simulink model "Lab3_Crazyflie_Task1"  (R2020a)
settings: Solver=FixedStepAuto  StartTime=0.0  StopTime=inf  MaxStep=0.1  RelTol=1e-3  EnableMultiTasking=on
PreLoadFcn:
  | % load parameters of the default quadrotor
  | disp('Quadrotor parameters loaded by PreLoadFcn')
  | mdl_quadrotor
undefined symbols (not defined in the file or in its folder): Pitch, Roll, rot2, Thrust, YawRate
libraries: robotlib x3, simulink x2
settings Model: Creator=corkep  LastModifiedBy=Pablo
settings DataIOCC: LimitDataPoints=on  ReturnWorkspaceOutputs=off
settings OptimizationCC: EnhancedBackFolding=on  PassReuseOutputArgsAs=Individual arguments  ExpressionDepthLimit=2147483647  ZeroExternalMemoryAtStartup=off  ZeroInternalMemoryAtStartup=off  MaxStackSize=64  OptimizeBlockOrder=speed  DifferentSizesBufferReuse=on  OptimizationCustomize=off  EfficientTunableParamExpr=on
settings DebuggingCC: UnderspecifiedInitializationDetection=Classic  MergeDetectMultiDrivingBlocksExec=none  SolverPrmCheckMsg=warning  ParameterTunabilityLossMsg=error  AllowSymbolicDim=off  StateNameClashWarn=warning  SFUnexpectedBacktrackingDiag=warning  SFNoUnconditionalDefaultTransitionDiag=warning  SFExecutionAtInitializationDiag=none  ArithmeticOperatorsInVariantConditions=warning
settings HardwareCC: ProdBitPerPointer=32  ProdBitPerSizeT=32  ProdBitPerPtrDiffT=32  ProdLargestAtomicFloat=None  ProdIntDivRoundTo=Undefined  ProdEndianess=Unspecified  ProdWordSize=32  ProdHWDeviceType=Generic->Unspecified (assume 32-bit Generic)  UseEmbeddedCoderFeatures=off
settings ModelReferenceCC: PropagateSignalLabelsOutOfModel=off
settings SFSimCC: SimUseLocalCustomCode=off  MATLABDynamicMemAlloc=off  CustomCodeUndefinedFunction=UseInterfaceOnly
settings RTWCC: SystemTargetFile=ert.tlc  HardwareBoard=Robot Operating System (ROS)  TemplateMakefile=ert_default_tmf  RTWUseLocalCustomCode=off  Toolchain=Catkin  TargetLang=C++
settings CodeAppCC: ForceParamTrailComments=on  IgnoreCustomStorageClasses=off  OperatorAnnotations=on  SimulinkDataObjDesc=on  SFDataObjDesc=on  InsertBlockDesc=on
settings ERTTargetCC: SupportNonInlinedSFcns=on
settings ConfigComp: CovMetricSettings=dw  CovHtmlReporting=on  CovSaveCumulativeToWorkspaceVar=on  CovSaveSingleToWorkspaceVar=on  CovExternalEMLEnable=off  CovSFcnEnable=off

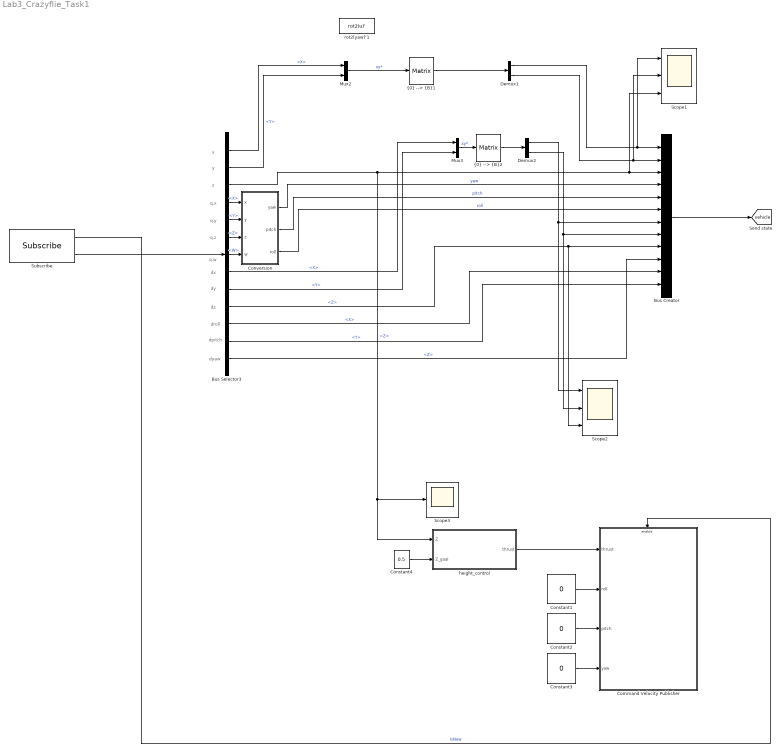
== system Lab3_Crazyflie_Task1 ==
  note: dyaw
  note: dpitch
  note: droll
  note: dz
  note: dy
  note: dx
  note: x
  note: y
  note: z
  note: q.x
  note: q.y
  note: q.z
  note: q.w
  Bus Creator : BusCreator  Inputs=12
  Bus Selector3 : BusSelector  OutputSignals=Pose.Pose.Position.X,Pose.Pose.Position.Y,Pose.Pose.Position.Z,Pose.Pose.Orientation.X,Pose.Pose.Orientation.Y,Pose.Pose.Orientation.Z,Pose.Pose.Orientation.W,Twist.Twist.Linear.X,Twist.Twist.Linear.Y,Twist.Twist.Linear.Z,Twist.Twist.Angular.X,Twist.Twist.Angular.Y,Twist.Twist.Angular.Z
  Command Velocity Publisher : Subsystem
  Constant1 : Constant  Value=0
  Constant2 : Constant  Value=0
  Constant3 : Constant  Value=0
  Constant4 : Constant  Value=0.5
  Conversion : MATLAB Function  TreatAsAtomicUnit=on
  Demux1 : Demux  Outputs=2
  Demux2 : Demux  Outputs=2
  Mux2 : Mux  Inputs=2
  Mux3 : Mux  Inputs=2
  Scope1 : Scope  NumInputPorts=3
  Scope2 : Scope  NumInputPorts=3
  Scope3 : Scope
  Subscribe : robotlib/Subscribe  topicSource=Select from ROS network  topic=/crazyflie2/ground_truth/odometry  messageType=nav_msgs/Odometry  sampleTime=-1  messageQueueLength=51
  height_control : Subsystem
  rot2(yaw)'1 : MATLABFcn  MATLABFcn=rot2(u)'  OutputDimensions=[2 2]  Output1D=off
  "{0} --> {B}1" : Product  Inputs=1  Multiplication=Matrix(*)  RndMeth=Zero
  "{0} --> {B}2" : Product  Inputs=1  Multiplication=Matrix(*)  RndMeth=Zero
  tag scope: vehicle=global
  wires:
  Bus Selector3/11 -> Bus Creator/11  "<X>"
  Bus Selector3/13 -> Bus Creator/10  "<Z>"
  Conversion/1(yaw) -> Bus Creator/4  "yaw"
  Bus Selector3/10 -> Bus Creator/9, Scope2/3  "<Z>"
  Bus Selector3/9 -> Mux3/2  "<Y>"
  Bus Selector3/8 -> Mux3/1  "<X>"
  Conversion/2(pitch) -> Bus Creator/5  "pitch"
  Bus Selector3/3 -> height_control/1(Z), Scope3/1, Scope1/3, Bus Creator/3  "<Z>"
  Bus Creator/1 -> [vehicle]
  Bus Selector3/12 -> Bus Creator/12  "<Y>"
  Conversion/3(roll) -> Bus Creator/6  "roll"
  Subscribe/2 -> Bus Selector3/1
  Bus Selector3/4 -> Conversion/1(x)  "<X>"
  Bus Selector3/5 -> Conversion/2(y)  "<Y>"
  Bus Selector3/6 -> Conversion/3(z)  "<Z>"
  Bus Selector3/7 -> Conversion/4(w)  "<W>"
  Subscribe/1 -> Command Velocity Publisher/Enable  "IsNew"
  Mux2/1 -> "{0} --> {B}1"/1  "xy*"
  "{0} --> {B}1"/1 -> Demux1/1
  "{0} --> {B}2"/1 -> Demux2/1
  Mux3/1 -> "{0} --> {B}2"/1  "xy*"
  Demux1/1 -> Bus Creator/1, Scope1/1
  Demux1/2 -> Bus Creator/2, Scope1/2
  Bus Selector3/1 -> Mux2/1  "<X>"
  Bus Selector3/2 -> Mux2/2  "<Y>"
  Demux2/1 -> Bus Creator/7, Scope2/1
  Demux2/2 -> Bus Creator/8, Scope2/2
  height_control/1(thrust) -> Command Velocity Publisher/1(thrust)
  Constant1/1 -> Command Velocity Publisher/2(roll)
  Constant2/1 -> Command Velocity Publisher/3(pitch)
  Constant3/1 -> Command Velocity Publisher/4(yaw)
  Constant4/1 -> height_control/2(Z_goal)

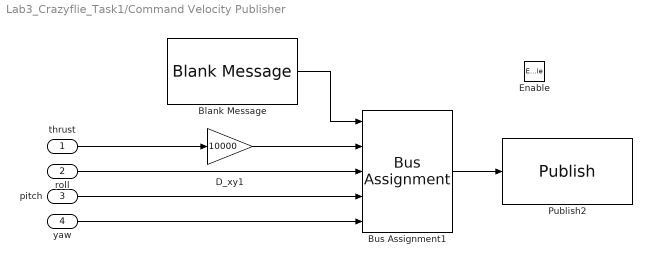
== system Lab3_Crazyflie_Task1/Command Velocity Publisher ==
  thrust : Inport
  roll : Inport  Port=2
  pitch : Inport  Port=3
  yaw : Inport  Port=4
  Enable : EnablePort
  Blank Message : robotlib/Blank Message  messageClass=Message  entityType=mav_msgs/RollPitchYawrateThrustCrazyflie  messageType=mav_msgs/RollPitchYawrateThrustCrazyflie  SampleTime=inf
  Bus Assignment1 : BusAssignment  DialogController=Simulink.DDGSource_BusAssignment  AssignedSignals=Thrust,Roll,Pitch,YawRate
  D_xy1 : Gain  Gain=10000
  Publish2 : robotlib/Publish  topicSource=Select from ROS network  topic=/crazyflie2/command/roll_pitch_yawrate_thrust  messageType=mav_msgs/RollPitchYawrateThrustCrazyflie  messageQueueLength=105
  wires:
  Blank Message/1 -> Bus Assignment1/1
  Bus Assignment1/1 -> Publish2/1
  thrust/1 -> D_xy1/1
  roll/1 -> Bus Assignment1/3
  pitch/1 -> Bus Assignment1/4
  yaw/1 -> Bus Assignment1/5
  D_xy1/1 -> Bus Assignment1/2

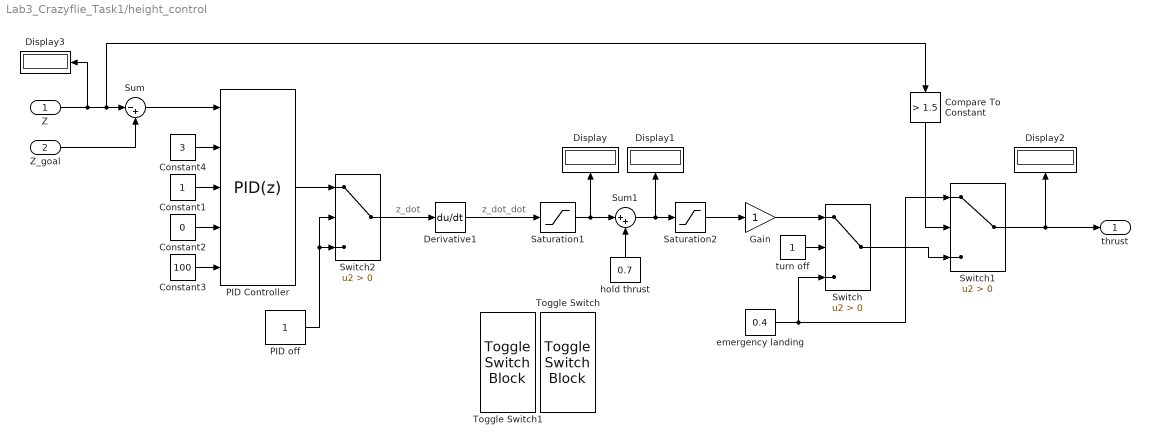
== system Lab3_Crazyflie_Task1/height_control ==
  note: z_dot
  note: z_dot_dot
  Z : Inport
  Z_goal : Inport  Port=2
  Compare To Constant : simulink/Logic and Bit Operations/Compare To Constant  relop=>  const=1.5  OutDataTypeStr=boolean
  Constant1 : Constant
  Constant2 : Constant  Value=0
  Constant3 : Constant  Value=100
  Constant4 : Constant  Value=3
  Derivative1 : Derivative
  Display{,1..3} (4 alike) : Display
  Gain : Gain
  PID Controller : simulink/Continuous/PID Controller  Controller=PID  Form=Parallel  TimeDomain=Discrete-time  UseExternalTs=off  SampleTime=-1  IntegratorMethod=Forward Euler  FilterMethod=Forward Euler  ControllerParametersSource=external  P=1  I=0  D=0  UseFilter=on  N=1000  TunerSelectOption=Transfer Function Based (PID Tuner App)  InitialConditionSource=internal  InitialConditionForIntegrator=0  InitialConditionForFilter=0  DifferentiatorICPrevScaledInput=0  ExternalReset=none  TrackingMode=off  Kt=1  LimitOutput=off  UpperSaturationLimit=inf  LowerSaturationLimit=-inf  LinearizeAsGain=on  AntiWindupMode=none  Kb=1  POutMin=[]  POutMax=[]  IOutMin=[]  IOutMax=[]  DOutMin=[]  DOutMax=[]  NOutMin=[]  NOutMax=[]  SumOutMin=[]  SumOutMax=[]  SaturationOutMin=[]  SaturationOutMax=[]  PParamMin=[]  PParamMax=[]  IParamMin=[]  IParamMax=[]  DParamMin=[]  DParamMax=[]  NParamMin=[]  NParamMax=[]  KbParamMin=[]  KbParamMax=[]  KtParamMin=[]  KtParamMax=[]  KbOutMin=[]  KbOutMax=[]  KtOutMin=[]  KtOutMax=[]  IntegratorOutMin=[]  IntegratorOutMax=[]  FilterOutMin=[]  FilterOutMax=[]  SumI1OutMin=[]  SumI1OutMax=[]  SumI2OutMin=[]  SumI2OutMax=[]  SumI3OutMin=[]  SumI3OutMax=[]  SumI4OutMin=[]  SumI4OutMax=[]  SumDOutMin=[]  SumDOutMax=[]  DifferentiatorOutMin=[]  DifferentiatorOutMax=[]  FilterDiffOutCoefMin=[]  FilterDiffOutCoefMax=[]  ReciprocalOutMin=[]  ReciprocalOutMax=[]  SumDenOutMin=[]  SumDenOutMax=[]  SumNumOutMin=[]  SumNumOutMax=[]  DivideOutMin=[]  DivideOutMax=[]  UdiffTsProdOutMin=[]  UdiffTsProdOutMax=[]  NTsProdOutMin=[]  NTsProdOutMax=[]  UintegralTsProdOutMin=[]  UintegralTsProdOutMax=[]  UngainTsProdOutMin=[]  UngainTsProdOutMax=[]  IntegratorContinuousStateAttributes=''  IntegratorStateMustResolveToSignalObject=off  IntegratorRTWStateStorageClass=Auto  FilterContinuousStateAttributes=''  FilterStateMustResolveToSignalObject=off  FilterRTWStateStorageClass=Auto  ParallelPVariant=ExternalParameters  IdealPVariant=Disabled  IVariant=ExternalParameters  DVariant=ExternalParameters  IntegratorVariant=Discrete  SatVariant=Disabled  AWVariant=Passthrough  PCopyVariant=Disabled  TRVariant=Disabled  FdbkBlocksVariant=Forward  IdealPFdbkVariant=Disabled  SatFdbkVariant=Disabled  DerivativeFilterVariant=ForwardEulerFilter  NVariant=ExternalParameters  NCopyVariant=Disabled  FilterICVariant=InternalICsFilter  IntegratorICVariant=InternalICs  ExternalResetVariant=Disabled  TRSumVariant=Passthrough  SumFdbkVariant=Disabled  SumVariant=Sum_PID  TsampFilterVariant=InternalTs  TsampNgainVariant=Passthrough  TsampIntegralVariant=Passthrough
  PID off : Constant
  Saturation1 : Saturate  UpperLimit=0.1  LowerLimit=-0.1
  Saturation2 : Saturate  UpperLimit=1  LowerLimit=0
  Sum : Sum  Inputs=|-+
  Sum1 : Sum  Inputs=|++
  Switch : Switch  Criteria=u2 > Threshold
  Switch1 : Switch  Criteria=u2 > Threshold
  Switch2 : Switch  Criteria=u2 > Threshold
  Toggle Switch : ToggleSwitchBlock
      settings: Values={{'Off', 'On'}, [0 1]}
  Toggle Switch1 : ToggleSwitchBlock
      settings: Values={{'Off', 'On'}, [0 1]}
  emergency landing : Constant  Value=0.4
  hold thrust : Constant  Value=0.7
  turn off : Constant
  thrust : Outport
  wires:
  Z/1 -> Compare To Constant/1, Sum/1, Display3/1
  Constant4/1 -> PID Controller/2
  Constant1/1 -> PID Controller/3
  Constant2/1 -> PID Controller/4
  Constant3/1 -> PID Controller/5
  hold thrust/1 -> Sum1/2
  Z_goal/1 -> Sum/2
  Saturation1/1 -> Sum1/1, Display/1
  Sum/1 -> PID Controller/1
  turn off/1 -> Switch/2
  Sum1/1 -> Saturation2/1, Display1/1
  Compare To Constant/1 -> Switch1/2
  emergency landing/1 -> Switch/3, Switch1/1
  Switch/1 -> Switch1/3
  Switch1/1 -> thrust/1, Display2/1
  PID off/1 -> Switch2/2, Switch2/3
  PID Controller/1 -> Switch2/1
  Saturation2/1 -> Gain/1
  Switch2/1 -> Derivative1/1
  Derivative1/1 -> Saturation1/1
  Gain/1 -> Switch/1

== matlab function Lab3_Crazyflie_Task1/Conversion ==
  data: yaw output; x input; y input; z input; w input; pitch output; roll output
function [yaw,pitch,roll]  = quat2eul(x,y,z,w)
%#codegen

% Convert the quaternion to a yaw angle (zyx euler angle)
eul = quat2eul([w,x,y,z]);
yaw = eul(1);
roll = eul(3);
pitch = eul(2);

end
